simulink model "gm_HDLRx_vs"  (R2024a)
settings: Solver=FixedStepDiscrete  StartTime=0.0  StopTime=stopTime  RelTol=1e-3
undefined symbols (not defined in the file or in its folder): channelBitsPerSubcarrier, channelCyclicPrefixLen, channelOFDMSamples, channelScramblerInit, clk, clk_enable, decimatorDelay, decimatorFilter, fPHY, fs, headerBitsPerFec, headerBitsPerSubcarrier, headerCyclicPrefixLen, headerOFDMSamples, headerScramblerInit, lowerbound, N, numDataCarriers, payloadBitsPerFec, payloadScramblerInit, preambleBitsPerSubcarrier, preambleCyclicPrefixLen, preambleFirstPartOFDMSamples, preambleScramblerInit, preambleSecondPartOFDMSamples, QAM, reset_x, upperbound
libraries: hdlsllib x133, hdlmdlgenlib x132, simulink x8, whdlutilities x8, whdlmod x4, dspsrcs4 x2, whdledac x2, commhdlcrc x1, dsphdlfiltering2 x1, dsphdlsigops2 x1, vivadosimlib x1, HDL_ieee_8021513 x1
(part 3 of 4)

== system gm_HDLRx_vs/full_rx/h_rx_full/h_separate/Compare To Constant ==
  u : Inport  OutDataTypeStr=fixdt(0, 5, 0)  SampleTime=8e-08
  Compare : RelationalOperator  Operator===  OutDataTypeStr=boolean
  Constant : Constant  DisableCoverage=on  Value=const  OutDataTypeStr=fixdt(0, 5, 0)  SampleTime=-1
  y : Outport  SampleTime=8e-08
  wires:
  Constant/1 -> Compare/2
  Compare/1 -> y/1
  u/1 -> Compare/1

== system gm_HDLRx_vs/full_rx/h_rx_full/h_separate/Compare To Constant1 ==
  u : Inport  OutDataTypeStr=fixdt(0, 5, 0)  SampleTime=8e-08
  Compare : RelationalOperator  Operator===  OutDataTypeStr=boolean
  Constant : Constant  DisableCoverage=on  Value=const  OutDataTypeStr=fixdt(0, 5, 0)  SampleTime=-1
  y : Outport  SampleTime=8e-08
  wires:
  Constant/1 -> Compare/2
  Compare/1 -> y/1
  u/1 -> Compare/1

== system gm_HDLRx_vs/full_rx/h_rx_full/h_separate/Compare To Constant2 ==
  u : Inport  OutDataTypeStr=fixdt(0, 5, 0)  SampleTime=8e-08
  Compare : RelationalOperator  Operator===  OutDataTypeStr=boolean
  Constant : Constant  DisableCoverage=on  Value=const  OutDataTypeStr=fixdt(0, 5, 0)  SampleTime=-1
  y : Outport  SampleTime=8e-08
  wires:
  Constant/1 -> Compare/2
  Compare/1 -> y/1
  u/1 -> Compare/1

== system gm_HDLRx_vs/full_rx/h_rx_full/h_separate/Compare To Constant3 ==
  u : Inport  OutDataTypeStr=fixdt(0, 5, 0)  SampleTime=8e-08
  Compare : RelationalOperator  Operator===  OutDataTypeStr=boolean
  Constant : Constant  DisableCoverage=on  Value=const  OutDataTypeStr=fixdt(0, 5, 0)  SampleTime=-1
  y : Outport  SampleTime=8e-08
  wires:
  Constant/1 -> Compare/2
  Compare/1 -> y/1
  u/1 -> Compare/1

== system gm_HDLRx_vs/full_rx/h_rx_full/h_separate/Compare To Constant4 ==
  u : Inport  OutDataTypeStr=fixdt(0, 5, 0)  SampleTime=8e-08
  Compare : RelationalOperator  Operator===  OutDataTypeStr=boolean
  Constant : Constant  DisableCoverage=on  Value=const  OutDataTypeStr=fixdt(0, 5, 0)  SampleTime=-1
  y : Outport  SampleTime=8e-08
  wires:
  Constant/1 -> Compare/2
  Compare/1 -> y/1
  u/1 -> Compare/1

== system gm_HDLRx_vs/full_rx/h_rx_full/h_separate/Compare To Constant5 ==
  u : Inport  OutDataTypeStr=fixdt(0, 5, 0)  SampleTime=8e-08
  Compare : RelationalOperator  Operator===  OutDataTypeStr=boolean
  Constant : Constant  DisableCoverage=on  Value=const  OutDataTypeStr=fixdt(0, 5, 0)  SampleTime=-1
  y : Outport  SampleTime=8e-08
  wires:
  Constant/1 -> Compare/2
  Compare/1 -> y/1
  u/1 -> Compare/1

== system gm_HDLRx_vs/full_rx/h_rx_full/h_separate/Compare To Constant6 ==
  u : Inport  OutDataTypeStr=fixdt(0, 5, 0)  SampleTime=8e-08
  Compare : RelationalOperator  Operator===  OutDataTypeStr=boolean
  Constant : Constant  DisableCoverage=on  Value=const  OutDataTypeStr=fixdt(0, 5, 0)  SampleTime=-1
  y : Outport  SampleTime=8e-08
  wires:
  Constant/1 -> Compare/2
  Compare/1 -> y/1
  u/1 -> Compare/1

== system gm_HDLRx_vs/full_rx/rx_demodulator_full/constellation_descrambler/rising_edge_detector ==
  In : Inport  OutDataTypeStr=boolean  SampleTime=2e-08
  Delay2 : Delay  DelayLength=1  InitialCondition=0  UseCircularBuffer=on
  Logical Operator1 : Logic  IconShape=distinctive  AllPortsSameDT=off  OutDataTypeStr=boolean
  Logical Operator2 : Logic  Operator=NOT  IconShape=distinctive  AllPortsSameDT=off  OutDataTypeStr=boolean
  Out : Outport  SampleTime=2e-08
  wires:
  Logical Operator2/1 -> Logical Operator1/2
  Logical Operator1/1 -> Out/1
  Delay2/1 -> Logical Operator2/1
  In/1 -> Delay2/1, Logical Operator1/1

== system gm_HDLRx_vs/full_rx/rx_demodulator_full/constellation_descrambler/rotate_-90 ==
  data_in : Inport  OutDataTypeStr=fixdt(1, 24, 12)  PortDimensions=1  SampleTime=2e-08
      settings: SignalType=complex
  valid_in : Inport  Port=2  OutDataTypeStr=boolean  PortDimensions=1  SampleTime=2e-08
  s1_in : Inport  Port=3  OutDataTypeStr=boolean  PortDimensions=1  SampleTime=2e-08
  s2_in : Inport  Port=4  OutDataTypeStr=boolean  PortDimensions=1  SampleTime=2e-08
  Delay : Delay  InitialCondition=0  UseCircularBuffer=on
  Delay1 : Delay  InitialCondition=0  UseCircularBuffer=on
  Delay2 : Delay  DelayLength=1  InitialCondition=0  UseCircularBuffer=on
  Delay3 : Delay  DelayLength=1  InitialCondition=0  UseCircularBuffer=on
  rotate_-90 : Subsystem
  data_out : Outport  SampleTime=2e-08  VectorParamsAs1DForOutWhenUnconnected=off
  valid_out : Outport  Port=2  SampleTime=2e-08  VectorParamsAs1DForOutWhenUnconnected=off
  wires:
  rotate_-90/1(data_out) -> Delay2/1
  Delay3/1 -> valid_out/1
  Delay2/1 -> data_out/1
  Delay1/1 -> Delay3/1
  Delay/1 -> rotate_-90/3(data_in)
  s2_in/1 -> rotate_-90/1(s2)
  s1_in/1 -> rotate_-90/2(s1)
  valid_in/1 -> Delay1/1
  data_in/1 -> Delay/1

== system gm_HDLRx_vs/full_rx/rx_demodulator_full/constellation_descrambler/sync_constellation_scrambler ==
  new_ofdm_symbol : Inport  OutDataTypeStr=boolean  SampleTime=2e-08
  init : Inport  Port=2  OutDataTypeStr=boolean  PortDimensions=[13]  SampleTime=2e-08
  valid_in : Inport  Port=3  OutDataTypeStr=boolean  SampleTime=2e-08
  Rate Transition : RateTransition  OutPortSampleTime=1/fPHY
  Rate Transition1 : RateTransition  OutPortSampleTime=1/fPHY
  Rate Transition2 : RateTransition  OutPortSampleTime=1/(2*fPHY)
  Rate Transition3 : RateTransition  OutPortSampleTime=1/(2*fPHY)
  Rate Transition4 : RateTransition  OutPortSampleTime=1/(2*fPHY)
  Synchronous constellation scrambler : Subsystem
  s1 : Outport  SampleTime=2e-08
  s2 : Outport  Port=2  SampleTime=2e-08
  wires:
  Synchronous constellation scrambler/2(s2_out) -> Rate Transition/1
  Synchronous constellation scrambler/1(s1_out) -> Rate Transition1/1
  Rate Transition4/1 -> Synchronous constellation scrambler/1(valid_in)
  Rate Transition3/1 -> Synchronous constellation scrambler/2(init)
  Rate Transition2/1 -> Synchronous constellation scrambler/3(new_ofdm_symbol)
  Rate Transition1/1 -> s1/1
  Rate Transition/1 -> s2/1
  valid_in/1 -> Rate Transition4/1
  init/1 -> Rate Transition3/1
  new_ofdm_symbol/1 -> Rate Transition2/1

== system gm_HDLRx_vs/full_rx/rx_demodulator_full/decimator/rising_edge_detector ==
  In : Inport  OutDataTypeStr=boolean  SampleTime=1e-08
  Delay2 : Delay  DelayLength=1  InitialCondition=0  UseCircularBuffer=on
  Logical Operator1 : Logic  IconShape=distinctive  AllPortsSameDT=off  OutDataTypeStr=boolean
  Logical Operator2 : Logic  Operator=NOT  IconShape=distinctive  AllPortsSameDT=off  OutDataTypeStr=boolean
  Out : Outport  SampleTime=1e-08
  wires:
  Logical Operator2/1 -> Logical Operator1/2
  Logical Operator1/1 -> Out/1
  Delay2/1 -> Logical Operator2/1
  In/1 -> Delay2/1, Logical Operator1/1

== system gm_HDLRx_vs/full_rx/rx_demodulator_full/downshifter/digital_carrier_receiver ==
  dataIn : Inport  OutDataTypeStr=fixdt(1, 16, 12)  PortDimensions=1  SampleTime=1e-08
  ncoIn : Inport  Port=2  OutDataTypeStr=fixdt(1, 16, 12)  PortDimensions=1  SampleTime=1e-08
      settings: SignalType=complex
  Complex to Real-Imag : ComplexToRealImag
  Constant : Constant  Value=2  OutDataTypeStr=fixdt(1, 16, 12)  SampleTime=-1
  Delay{,1..4} (5 alike) : Delay  InitialCondition=0  UseCircularBuffer=on
  Product : Product  OutDataTypeStr=fixdt(1, 16, 12)
  Product1 : Product  InputSameDT=on  OutDataTypeStr=fixdt(1, 16, 12)
  Product2 : Product  OutDataTypeStr=fixdt(1, 16, 12)
  Real-Imag to Complex : RealImagToComplex
  Unary Minus : UnaryMinus
  data_out : Outport  SampleTime=1e-08  VectorParamsAs1DForOutWhenUnconnected=off
  wires:
  Unary Minus/1 -> Delay3/1
  Real-Imag to Complex/1 -> data_out/1
  Product2/1 -> Delay4/1
  Product1/1 -> Delay2/1
  Product/1 -> Delay/1
  Delay4/1 -> Real-Imag to Complex/2
  Delay3/1 -> Product2/1
  Delay2/1 -> Complex to Real-Imag/1
  Delay1/1 -> Product/1
  Delay/1 -> Real-Imag to Complex/1
  Constant/1 -> Product1/1
  Complex to Real-Imag/2 -> Product2/2
  Complex to Real-Imag/1 -> Product/2
  ncoIn/1 -> Product1/2
  dataIn/1 -> Delay1/1, Unary Minus/1

== system gm_HDLRx_vs/full_rx/rx_demodulator_full/downshifter/rising_edge_detector ==
  In : Inport  OutDataTypeStr=boolean  SampleTime=1e-08
  Delay2 : Delay  DelayLength=1  InitialCondition=0  UseCircularBuffer=on
  Logical Operator1 : Logic  IconShape=distinctive  AllPortsSameDT=off  OutDataTypeStr=boolean
  Logical Operator2 : Logic  Operator=NOT  IconShape=distinctive  AllPortsSameDT=off  OutDataTypeStr=boolean
  Out : Outport  SampleTime=1e-08
  wires:
  Logical Operator2/1 -> Logical Operator1/2
  Logical Operator1/1 -> Out/1
  Delay2/1 -> Logical Operator2/1
  In/1 -> Delay2/1, Logical Operator1/1

== system gm_HDLRx_vs/full_rx/rx_demodulator_full/ofdm_rx_counter/falling_edge_detector1 ==
  in : Inport  OutDataTypeStr=boolean  SampleTime=2e-08
  Delay : Delay  DelayLength=1  InitialCondition=0  UseCircularBuffer=on
  Logical Operator : Logic  IconShape=distinctive  AllPortsSameDT=off  OutDataTypeStr=boolean
  Logical Operator1 : Logic  Operator=NOT  IconShape=distinctive  AllPortsSameDT=off  OutDataTypeStr=boolean
  out : Outport  SampleTime=2e-08
  wires:
  Logical Operator1/1 -> Logical Operator/1
  Logical Operator/1 -> out/1
  Delay/1 -> Logical Operator/2
  in/1 -> Delay/1, Logical Operator1/1

== system gm_HDLRx_vs/full_rx/rx_demodulator_full/ofdm_rx_counter/rising_edge_detector1 ==
  In : Inport  OutDataTypeStr=boolean  SampleTime=2e-08
  Delay2 : Delay  DelayLength=1  InitialCondition=0  UseCircularBuffer=on
  Logical Operator1 : Logic  IconShape=distinctive  AllPortsSameDT=off  OutDataTypeStr=boolean
  Logical Operator2 : Logic  Operator=NOT  IconShape=distinctive  AllPortsSameDT=off  OutDataTypeStr=boolean
  Out : Outport  SampleTime=2e-08
  wires:
  Logical Operator2/1 -> Logical Operator1/2
  Logical Operator1/1 -> Out/1
  Delay2/1 -> Logical Operator2/1
  In/1 -> Delay2/1, Logical Operator1/1

== system gm_HDLRx_vs/full_rx/rx_demodulator_full/ofdm_separator/Real Divide HDL Optimized ==
  num : Inport  OutDataTypeStr=fixdt(0, 24, 0)  SampleTime=2e-08
  den : Inport  Port=2  OutDataTypeStr=uint16  SampleTime=2e-08
  validIn : Inport  Port=3  OutDataTypeStr=boolean  SampleTime=2e-08
  Delay17 : Delay  DelayLength=1
  ForEach - Real Divide_instance1 : Subsystem
  Reshape to original size : Subsystem
  Verify divide sizes : Subsystem
  y : Outport  SampleTime=2e-08
  wires:
  Verify divide sizes/2(num) -> ForEach - Real Divide_instance1/2(num)
  Verify divide sizes/1(den) -> ForEach - Real Divide_instance1/1(den)
  Reshape to original size/1(z) -> Delay17/1
  ForEach - Real Divide_instance1/1(y) -> Reshape to original size/1(y)
  Delay17/1 -> y/1
  validIn/1 -> ForEach - Real Divide_instance1/3(validIn)
  den/1 -> Verify divide sizes/1(denominator)
  num/1 -> Reshape to original size/2(u), Verify divide sizes/2(numerator)

== system gm_HDLRx_vs/full_rx/rx_demodulator_full/ofdm_separator/rising_edge_detector ==
  In : Inport  OutDataTypeStr=boolean  SampleTime=2e-08
  Delay2 : Delay  DelayLength=1  InitialCondition=0  UseCircularBuffer=on
  Logical Operator1 : Logic  IconShape=distinctive  AllPortsSameDT=off  OutDataTypeStr=boolean
  Logical Operator2 : Logic  Operator=NOT  IconShape=distinctive  AllPortsSameDT=off  OutDataTypeStr=boolean
  Out : Outport  SampleTime=2e-08
  wires:
  Logical Operator2/1 -> Logical Operator1/2
  Logical Operator1/1 -> Out/1
  Delay2/1 -> Logical Operator2/1
  In/1 -> Delay2/1, Logical Operator1/1

== system gm_HDLRx_vs/full_rx/rx_demodulator_full/qam_demod/to_12bit_integer ==
  1bit : Inport  OutDataTypeStr=fixdt(1, 28, 12)  PortDimensions=1  SampleTime=2e-08
  2bit : Inport  Port=2  OutDataTypeStr=fixdt(1, 28, 12)  PortDimensions=[2 1]  SampleTime=2e-08
  4bit : Inport  Port=3  OutDataTypeStr=fixdt(1, 28, 12)  PortDimensions=[4 1]  SampleTime=2e-08
  Constant{,1..2,12,14} (5 alike) : Constant  Value=0  OutDataTypeStr=fixdt(1, 28, 12)  SampleTime=2e-08
  concatenate : Concatenate  NumInputs=4  Mode=Multidimensional array
  concatenate1 : Concatenate  NumInputs=4  Mode=Multidimensional array
  t : Demux  Outputs=2
  1bit_out : Outport  SampleTime=2e-08
  2bit_out : Outport  Port=2  SampleTime=2e-08
  4bit_out : Outport  Port=3  SampleTime=2e-08
  wires:
  t/2 -> concatenate/4
  t/1 -> concatenate/3
  concatenate1/1 -> 1bit_out/1
  concatenate/1 -> 2bit_out/1
  Constant2/1 -> concatenate1/1
  Constant14/1 -> concatenate/1
  Constant12/1 -> concatenate/2
  Constant1/1 -> concatenate1/2
  Constant/1 -> concatenate1/3
  4bit/1 -> 4bit_out/1
  2bit/1 -> t/1
  1bit/1 -> concatenate1/4

== system gm_HDLRx_vs/full_rx/rx_payload_full/next_frame_to_ready_rx/rising_edge_detector ==
  In : Inport  OutDataTypeStr=boolean  SampleTime=1e-08
  Delay2 : Delay  DelayLength=1  InitialCondition=0  UseCircularBuffer=on
  Logical Operator1 : Logic  IconShape=distinctive  AllPortsSameDT=off  OutDataTypeStr=boolean
  Logical Operator2 : Logic  Operator=NOT  IconShape=distinctive  AllPortsSameDT=off  OutDataTypeStr=boolean
  Out : Outport  SampleTime=1e-08
  wires:
  Logical Operator2/1 -> Logical Operator1/2
  Logical Operator1/1 -> Out/1
  Delay2/1 -> Logical Operator2/1
  In/1 -> Delay2/1, Logical Operator1/1

== system gm_HDLRx_vs/full_rx/rx_payload_full/remove_tone_mapping/valid_to_ctrl ==
  validIn : Inport  OutDataTypeStr=boolean  SampleTime=1e-08
  Delay1 : Delay  DelayLength=1  InitialCondition=0  UseCircularBuffer=on
  Delay2 : Delay  DelayLength=1  InitialCondition=0  UseCircularBuffer=on
  Logical Operator : Logic  IconShape=distinctive  AllPortsSameDT=off  OutDataTypeStr=boolean
  Logical Operator1 : Logic  Operator=NOT  IconShape=distinctive  AllPortsSameDT=off  OutDataTypeStr=boolean
  Logical Operator2 : Logic  IconShape=distinctive  AllPortsSameDT=off  OutDataTypeStr=boolean
  Logical Operator3 : Logic  Operator=NOT  IconShape=distinctive  AllPortsSameDT=off  OutDataTypeStr=boolean
  Sample Control Bus Creator : whdlutilities/Sample Control Bus Creator
  ctrlOut : Outport  SampleTime=1e-08
  wires:
  Sample Control Bus Creator/1 -> ctrlOut/1
  Logical Operator3/1 -> Logical Operator2/2
  Logical Operator2/1 -> Sample Control Bus Creator/2
  Logical Operator1/1 -> Logical Operator/2
  Logical Operator/1 -> Sample Control Bus Creator/1
  Delay2/1 -> Logical Operator1/1
  Delay1/1 -> Sample Control Bus Creator/3, Delay2/1, Logical Operator/1, Logical Operator2/1
  validIn/1 -> Delay1/1, Logical Operator3/1

== system gm_HDLRx_vs/full_rx/rx_demodulator_full/constellation_descrambler/rotate_-90/rotate_-90 ==
  s2 : Inport  OutDataTypeStr=boolean  PortDimensions=1  SampleTime=2e-08
  s1 : Inport  Port=2  OutDataTypeStr=boolean  PortDimensions=1  SampleTime=2e-08
  data_in : Inport  Port=3  OutDataTypeStr=fixdt(1, 24, 12)  PortDimensions=1  SampleTime=2e-08
      settings: SignalType=complex
  Bit Concat : hdlsllib/Logic and Bit Operations/Bit Concat  numInputs=2
  Complex to Real-Imag : ComplexToRealImag
  Complex to Real-Imag1 : ComplexToRealImag
  Complex to Real-Imag2 : ComplexToRealImag
  Multiport Switch : MultiPortSwitch  DataPortOrder=Zero-based contiguous  Inputs=4  zeroidx=on  OutDataTypeStr=fixdt(1, 24, 12)  SaturateOnIntegerOverflow=off  InputSameDT=off
  Real-Imag to Complex : RealImagToComplex
  Real-Imag to Complex1 : RealImagToComplex
  Real-Imag to Complex2 : RealImagToComplex
  Unary Minus{,1..3} (4 alike) : UnaryMinus
  data_out : Outport  SampleTime=2e-08
  wires:
  Unary Minus3/1 -> Real-Imag to Complex/2
  Unary Minus2/1 -> Real-Imag to Complex2/1
  Unary Minus1/1 -> Real-Imag to Complex1/2
  Unary Minus/1 -> Real-Imag to Complex/1
  Real-Imag to Complex2/1 -> Multiport Switch/5
  Real-Imag to Complex1/1 -> Multiport Switch/3
  Real-Imag to Complex/1 -> Multiport Switch/4
  Multiport Switch/1 -> data_out/1
  Complex to Real-Imag2/2 -> Unary Minus2/1
  Complex to Real-Imag2/1 -> Real-Imag to Complex2/2
  Complex to Real-Imag1/2 -> Real-Imag to Complex1/1
  Complex to Real-Imag1/1 -> Unary Minus1/1
  Complex to Real-Imag/2 -> Unary Minus3/1
  Complex to Real-Imag/1 -> Unary Minus/1
  Bit Concat/1 -> Multiport Switch/1
  data_in/1 -> Complex to Real-Imag/1, Complex to Real-Imag1/1, Complex to Real-Imag2/1, Multiport Switch/2
  s1/1 -> Bit Concat/2
  s2/1 -> Bit Concat/1

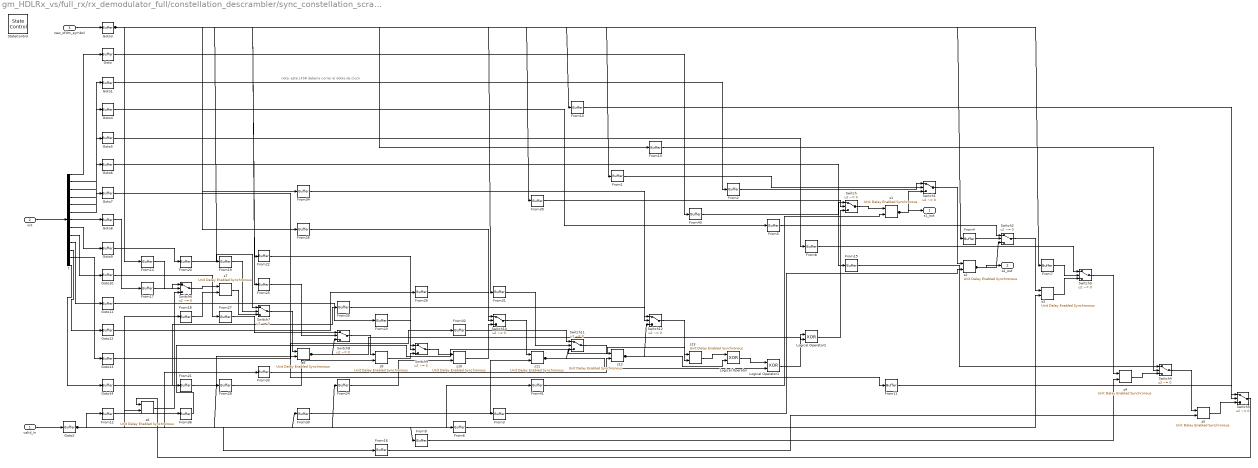
== system gm_HDLRx_vs/full_rx/rx_demodulator_full/constellation_descrambler/sync_constellation_scrambler/Synchronous constellation scrambler ==
  note: nota: este LFSR deberia correr al doble de clock
  valid_in : Inport  OutDataTypeStr=boolean  PortDimensions=1  SampleTime=1e-08
  init : Inport  Port=2  OutDataTypeStr=boolean  PortDimensions=[13]  SampleTime=1e-08
  new_ofdm_symbol : Inport  Port=3  OutDataTypeStr=boolean  PortDimensions=1  SampleTime=1e-08
  From{1..36,39..41} (39 alike) : hdlmdlgenlib/Buffer
  Goto{,1..14} (15 alike) : hdlmdlgenlib/Buffer
  Logical Operator : Logic  Operator=XOR  AllPortsSameDT=off  OutDataTypeStr=boolean  SampleTime=1e-08
  Logical Operator1 : Logic  Operator=XOR  AllPortsSameDT=off  OutDataTypeStr=boolean  SampleTime=1e-08
  Logical Operator2 : Logic  Operator=XOR  AllPortsSameDT=off  OutDataTypeStr=boolean  SampleTime=1e-08
  StateControl : StateControl  StateControl=Synchronous
  Switch{,1..12} (13 alike) : Switch  Criteria=u2 ~= 0  Threshold=double(0)  OutDataTypeStr=boolean  SampleTime=1e-08  SaturateOnIntegerOverflow=off  InputSameDT=off
  s{1..13} (13 alike) : hdlsllib/Discrete/Unit Delay Enabled Synchronous  InitialCondition=double(0)  SampleTime=-1
  t : Demux  Outputs=13
  s1_out : Outport  SampleTime=1e-08  VectorParamsAs1DForOutWhenUnconnected=off
  s2_out : Outport  Port=2  SampleTime=1e-08  VectorParamsAs1DForOutWhenUnconnected=off
  wires:
  t/13 -> Goto14/1
  t/12 -> Goto13/1
  t/11 -> Goto12/1
  t/10 -> Goto11/1
  t/9 -> Goto10/1
  t/8 -> Goto9/1
  t/7 -> Goto8/1
  t/6 -> Goto7/1
  t/5 -> Goto6/1
  t/4 -> Goto5/1
  t/3 -> Goto4/1
  t/2 -> Goto1/1
  t/1 -> Goto/1
  Goto5/1 -> From8/1
  Goto4/1 -> From5/1
  Goto/1 -> From40/1
  Goto14/1 -> From35/1
  Goto13/1 -> From32/1
  Goto12/1 -> From29/1
  Goto10/1 -> From27/1
  Goto11/1 -> From23/1
  Goto9/1 -> From20/1
  Goto1/1 -> From2/1
  Goto8/1 -> From17/1
  Goto6/1 -> From15/1
  Goto2/1 -> From12/1, From16/1, From18/1, From21/1, From24/1, From28/1, From3/1, From30/1, From33/1, From36/1, From41/1, From6/1, From9/1
  Goto7/1 -> From11/1
  Goto3/1 -> From1/1, From10/1, From13/1, From14/1, From19/1, From22/1, From25/1, From26/1, From31/1, From34/1, From39/1, From4/1, From7/1
  s9/1 -> Switch9/3
  s8/1 -> Logical Operator2/2, Switch8/3
  s7/1 -> Switch7/3
  s6/1 -> Switch6/3
  s5/1 -> Switch5/3
  s4/1 -> Switch4/3
  s3/1 -> Switch3/3
  s2/1 -> s2_out/1, Switch2/3
  s13/1 -> Logical Operator/1
  s12/1 -> Logical Operator/2, Switch12/3
  s11/1 -> Logical Operator1/2, Switch11/3
  s10/1 -> Switch10/3
  s1/1 -> s1_out/1, Switch1/3
  Switch9/1 -> s10/1
  Switch8/1 -> s9/1
  Switch7/1 -> s8/1
  Switch6/1 -> s7/1
  Switch5/1 -> s6/1
  Switch4/1 -> s5/1
  Switch3/1 -> s4/1
  Switch2/1 -> s3/1
  Switch12/1 -> s13/1
  Switch11/1 -> s12/1
  Switch10/1 -> s11/1
  Switch1/1 -> s2/1
  Switch/1 -> s1/1
  Logical Operator2/1 -> Switch/3
  Logical Operator1/1 -> Logical Operator2/1
  Logical Operator/1 -> Logical Operator1/1
  From9/1 -> s4/2
  From8/1 -> Switch3/1
  From7/1 -> Switch3/2
  From6/1 -> s3/2
  From5/1 -> Switch2/1
  From41/1 -> s1/2
  From40/1 -> Switch/1
  From4/1 -> Switch2/2
  From39/1 -> Switch/2
  From36/1 -> s13/2
  From35/1 -> Switch12/1
  From34/1 -> Switch12/2
  From33/1 -> s12/2
  From32/1 -> Switch11/1
  From31/1 -> Switch11/2
  From30/1 -> s11/2
  From3/1 -> s2/2
  From29/1 -> Switch10/1
  From28/1 -> s9/2
  From27/1 -> Switch8/1
  From26/1 -> Switch10/2
  From25/1 -> Switch8/2
  From24/1 -> s10/2
  From23/1 -> Switch9/1
  From22/1 -> Switch9/2
  From21/1 -> s8/2
  From20/1 -> Switch7/1
  From2/1 -> Switch1/1
  From19/1 -> Switch7/2
  From18/1 -> s7/2
  From17/1 -> Switch6/1
  From16/1 -> s5/2
  From15/1 -> Switch4/1
  From14/1 -> Switch6/2
  From13/1 -> Switch4/2
  From12/1 -> s6/2
  From11/1 -> Switch5/1
  From10/1 -> Switch5/2
  From1/1 -> Switch1/2
  new_ofdm_symbol/1 -> Goto3/1
  init/1 -> t/1
  valid_in/1 -> Goto2/1

== system gm_HDLRx_vs/full_rx/rx_demodulator_full/ofdm_separator/Real Divide HDL Optimized/ForEach - Real Divide_instance1 ==
  note: For Each
  den : Inport  OutDataTypeStr=uint16  PortDimensions=1  SampleTime=2e-08
  num : Inport  Port=2  OutDataTypeStr=fixdt(0, 24, 0)  PortDimensions=1  SampleTime=2e-08
  validIn : Inport  Port=3  OutDataTypeStr=boolean  PortDimensions=1  SampleTime=2e-08
  Delay{1,4,14..17,25..26} (8 alike) : Delay  DelayLength=1
  Delay{2,9..12,18} (6 alike) : Delay
  Divide by zero handler : Subsystem
  Divide real numerator by denominator : Subsystem
  MATLAB Function : Subsystem
  Normalize denominator : Subsystem  mask(Real Normalizer HDL Optimized){}
      mask help: fixed:emblib:RealNormalizerFullDescription
      mask Help: For internal use only. This feature is intentionally undocumented. Its behavior may change, or it may be removed in a future release.
      mask Display:
      | text(0.5,0.8,'u ~= 0','texmode','on','HorizontalAlignment','center')
      | text(0.5,0.6,'x = 2^e |u|','texmode','on','HorizontalAlignment','center')
      | text(0.5,0.4,'1 \leq x < 2','texmode','on','HorizontalAlignment','center')
      | text(0.5,0.2,'isNegative = u<0','texmode','on','HorizontalAlignment','center')
  Normalize numerator : Subsystem  mask(Real Normalizer HDL Optimized){}
      mask help: fixed:emblib:RealNormalizerFullDescription
      mask Help: For internal use only. This feature is intentionally undocumented. Its behavior may change, or it may be removed in a future release.
      mask Display:
      | text(0.5,0.8,'u ~= 0','texmode','on','HorizontalAlignment','center')
      | text(0.5,0.6,'x = 2^e |u|','texmode','on','HorizontalAlignment','center')
      | text(0.5,0.4,'1 \leq x < 2','texmode','on','HorizontalAlignment','center')
      | text(0.5,0.2,'isNegative = u<0','texmode','on','HorizontalAlignment','center')
  Shift and cast to output type : Subsystem  mask{OutputType=OutputType}
      mask prompts: OutputType "fixed:emblib:OutputPrototype"
  Switch : Switch  Criteria=u2 ~= 0  OutDataTypeStr=int16  SaturateOnIntegerOverflow=off  InputSameDT=off
  Unit Delay Enabled Synchronous : hdlsllib/Discrete/Unit Delay Enabled Synchronous  InitialCondition=0.0  SampleTime=-1
  Unit Delay Enabled Synchronous1 : hdlsllib/Discrete/Unit Delay Enabled Synchronous  InitialCondition=0.0  SampleTime=-1
  Unit Delay Enabled Synchronous2 : hdlsllib/Discrete/Unit Delay Enabled Synchronous  InitialCondition=0.0  SampleTime=-1
      settings: LibrarySourceBlock=|
      | embreciprocals/Real Divide HDL Optimized/ForEach - Real Divide/Unit Delay Enabled
      | Synchronous1
  Upcast Wordlength : Subsystem
  y : Outport  SampleTime=2e-08
  wires:
  Delay1/1 -> y/1
  Delay10/1 -> Divide real numerator by denominator/4(tDen)
  Delay11/1 -> Divide real numerator by denominator/6(isDenNegative)
  Delay12/1 -> Divide real numerator by denominator/7(validIn)
  Delay14/1 -> Normalize numerator/1(u)
  Delay15/1 -> Normalize numerator/2(validIn), Normalize denominator/2(validIn)
  Delay16/1 -> Divide real numerator by denominator/1(num)
  Delay17/1 -> Divide real numerator by denominator/2(tNum)
  Delay18/1 -> Divide real numerator by denominator/5(isNumNegative)
  Delay2/1 -> Switch/2
  Delay25/1 -> MATLAB Function/1(num)
  Delay26/1 -> MATLAB Function/2(t_num)
  Delay4/1 -> Normalize denominator/1(u)
  Delay9/1 -> Divide real numerator by denominator/3(den)
  Divide by zero handler/1(yOut) -> Switch/1
  Divide real numerator by denominator/4(validOut) -> Unit Delay Enabled Synchronous2/2, Unit Delay Enabled Synchronous1/2, Unit Delay Enabled Synchronous/2
  Divide real numerator by denominator/3(isDenZero) -> Unit Delay Enabled Synchronous2/1
  Divide real numerator by denominator/2(e) -> Unit Delay Enabled Synchronous1/1
  Divide real numerator by denominator/1(y) -> Unit Delay Enabled Synchronous/1
  MATLAB Function/2(t_num_out) -> Delay17/1
  MATLAB Function/1(num_out) -> Delay16/1
  Normalize denominator/4(validOut) -> Delay12/1
  Normalize denominator/3(isNegative) -> Delay11/1
  Normalize denominator/2(e) -> Delay10/1
  Normalize denominator/1(x) -> Delay9/1
  Normalize numerator/3(isNegative) -> Delay18/1
  Normalize numerator/2(e) -> Delay26/1
  Normalize numerator/1(x) -> Delay25/1
  Shift and cast to output type/1(y) -> Switch/3
  Switch/1 -> Delay1/1
  Unit Delay Enabled Synchronous/1 -> Shift and cast to output type/1(x), Divide by zero handler/1(yIn)
  Unit Delay Enabled Synchronous1/1 -> Shift and cast to output type/2(shiftValue)
  Unit Delay Enabled Synchronous2/1 -> Delay2/1
  Upcast Wordlength/2(v) -> Delay14/1
  Upcast Wordlength/1(u) -> Delay4/1
  validIn/1 -> Delay15/1
  num/1 -> Upcast Wordlength/2(y)
  den/1 -> Upcast Wordlength/1(x)

== system gm_HDLRx_vs/full_rx/rx_demodulator_full/ofdm_separator/Real Divide HDL Optimized/Reshape to original size ==
  y : Inport  OutDataTypeStr=int16  PortDimensions=1  SampleTime=2e-08
  u : Inport  Port=2  OutDataTypeStr=fixdt(0, 24, 0)  PortDimensions=1  SampleTime=2e-08
  embreciprocals_c11_Reshape_to_original_size : MATLAB Function  TreatAsAtomicUnit=on
      settings: LibrarySourceBlock=embreciprocals/Real Divide HDL Optimized/Reshape to original size
  z : Outport  SampleTime=2e-08
  wires:
  embreciprocals_c11_Reshape_to_original_size/1(z) -> z/1
  u/1 -> embreciprocals_c11_Reshape_to_original_size/2(u)
  y/1 -> embreciprocals_c11_Reshape_to_original_size/1(y)

== system gm_HDLRx_vs/full_rx/rx_demodulator_full/ofdm_separator/Real Divide HDL Optimized/Verify divide sizes ==
  denominator : Inport  OutDataTypeStr=uint16  PortDimensions=1  SampleTime=2e-08
  numerator : Inport  Port=2  OutDataTypeStr=fixdt(0, 24, 0)  PortDimensions=1  SampleTime=2e-08
  embreciprocals_c19_Verify_divide_sizes : MATLAB Function  TreatAsAtomicUnit=on
      settings: LibrarySourceBlock=embreciprocals/Real Divide HDL Optimized/Verify divide sizes
  den : Outport  SampleTime=2e-08
  num : Outport  Port=2  SampleTime=2e-08
  wires:
  embreciprocals_c19_Verify_divide_sizes/2(num) -> num/1
  embreciprocals_c19_Verify_divide_sizes/1(den) -> den/1
  numerator/1 -> embreciprocals_c19_Verify_divide_sizes/2(numerator)
  denominator/1 -> embreciprocals_c19_Verify_divide_sizes/1(denominator)

== system gm_HDLRx_vs/full_rx/rx_demodulator_full/ofdm_separator/Real Divide HDL Optimized/ForEach - Real Divide_instance1/Divide by zero handler ==
  yIn : Inport  OutDataTypeStr=fixdt(1, 25, 23)  SampleTime=2e-08
  Compare To Zero : Subsystem  mask(Compare To Zero){relop=>=, OutDataTypeStr=boolean, ZeroCross=on}
      mask prompts: relop "Simulink:masks:Operator_MP"; OutDataTypeStr "Simulink:masks:OutputDataType_MP"; ZeroCross "Simulink:masks:EnableZerocrossingDetection_MP"
      mask help: Simulink:masks:CompareToZero_MD
      mask init:
      | OutDataTypeStr = 'boolean';
      | ZeroCross = 'on';
      | blkName = 'HDLRx/full_rx/rx_demodulator_full/ofdm_separator/Real Divide HDL Optimized/ForEach - Real Divide/Divide by zero handler/Compare\nTo Zero';
      | relop = '>=';
      | setValue = 'boolean';
      mask TypeOptions relop: == | ~= | < | <= | >= | >
      mask TypeOptions OutDataTypeStr: Simulink:masks:uint8 | Simulink:masks:boolean
      mask Callback ZeroCross: sl('zeroCrossEnable', gcbh);
      mask Display: disp([relop,' 0'])
  Constant3 : Constant  Value=lowerbound(numerictype(OutputType))  OutDataTypeStr=OutputType  SampleTime=-1
  Constant4 : Constant  Value=upperbound(numerictype(OutputType))  OutDataTypeStr=OutputType  SampleTime=-1
  Delay13 : Delay  DelayLength=1
  Delay3 : Delay  DelayLength=1
  Switch : Switch  Criteria=u2 > Threshold  OutDataTypeStr=int16  SaturateOnIntegerOverflow=off  InputSameDT=off
  yOut : Outport  SampleTime=2e-08
  wires:
  yIn/1 -> Compare To Zero/1(u)
  Compare To Zero/1(y) -> Delay13/1
  Constant3/1 -> Switch/3
  Constant4/1 -> Switch/1
  Delay13/1 -> Switch/2
  Delay3/1 -> yOut/1
  Switch/1 -> Delay3/1

== system gm_HDLRx_vs/full_rx/rx_demodulator_full/ofdm_separator/Real Divide HDL Optimized/ForEach - Real Divide_instance1/Divide real numerator by denominator ==
  num : Inport  OutDataTypeStr=fixdt(1, 25, 23)  SampleTime=2e-08
  tNum : Inport  Port=2  OutDataTypeStr=fixdt(1, 33, 0)  SampleTime=2e-08
  den : Inport  Port=3  OutDataTypeStr=fixdt(1, 25, 23)  SampleTime=2e-08
  tDen : Inport  Port=4  OutDataTypeStr=int32  SampleTime=2e-08
  isNumNegative : Inport  Port=5  OutDataTypeStr=boolean  SampleTime=2e-08
  isDenNegative : Inport  Port=6  OutDataTypeStr=boolean  SampleTime=2e-08
  validIn : Inport  Port=7  OutDataTypeStr=boolean  SampleTime=2e-08
  normalizedCORDICDivide : Subsystem
  y : Outport  SampleTime=2e-08
  e : Outport  Port=2  SampleTime=2e-08
  isDenZero : Outport  Port=3  SampleTime=2e-08
  validOut : Outport  Port=4  SampleTime=2e-08
  wires:
  validIn/1 -> normalizedCORDICDivide/7(validIn)
  isDenNegative/1 -> normalizedCORDICDivide/6(isDenNegative)
  isNumNegative/1 -> normalizedCORDICDivide/5(isNumNegative)
  tDen/1 -> normalizedCORDICDivide/4(tDen)
  den/1 -> normalizedCORDICDivide/2(den)
  tNum/1 -> normalizedCORDICDivide/3(tNum)
  num/1 -> normalizedCORDICDivide/1(num)
  normalizedCORDICDivide/4(validOut) -> validOut/1
  normalizedCORDICDivide/3(isDenZeroOut) -> isDenZero/1
  normalizedCORDICDivide/2(t) -> e/1
  normalizedCORDICDivide/1(y) -> y/1

== system gm_HDLRx_vs/full_rx/rx_demodulator_full/ofdm_separator/Real Divide HDL Optimized/ForEach - Real Divide_instance1/MATLAB Function ==
  num : Inport  OutDataTypeStr=fixdt(1, 25, 23)  PortDimensions=1  SampleTime=2e-08
  t_num : Inport  Port=2  OutDataTypeStr=int32  PortDimensions=1  SampleTime=2e-08
  embreciprocals_c13_MATLAB_Function : MATLAB Function  TreatAsAtomicUnit=on
      settings: LibrarySourceBlock=embreciprocals/Real Divide HDL Optimized/ForEach - Real Divide/MATLAB Function
  num_out : Outport  SampleTime=2e-08
  t_num_out : Outport  Port=2  SampleTime=2e-08
  wires:
  embreciprocals_c13_MATLAB_Function/2(t_num_out) -> t_num_out/1
  embreciprocals_c13_MATLAB_Function/1(num_out) -> num_out/1
  t_num/1 -> embreciprocals_c13_MATLAB_Function/2(t_num)
  num/1 -> embreciprocals_c13_MATLAB_Function/1(num)

== system gm_HDLRx_vs/full_rx/rx_demodulator_full/ofdm_separator/Real Divide HDL Optimized/ForEach - Real Divide_instance1/Normalize denominator ==
  u : Inport  OutDataTypeStr=fixdt(1, 25, 8)  SampleTime=2e-08
  validIn : Inport  Port=2  OutDataTypeStr=boolean  SampleTime=2e-08
  positiveRealNormalizer : Subsystem
  x : Outport  SampleTime=2e-08
  e : Outport  Port=2  SampleTime=2e-08
  isNegative : Outport  Port=3  SampleTime=2e-08
  validOut : Outport  Port=4  SampleTime=2e-08
  wires:
  validIn/1 -> positiveRealNormalizer/2(validIn)
  u/1 -> positiveRealNormalizer/1(u)
  positiveRealNormalizer/4(validOut) -> validOut/1
  positiveRealNormalizer/3(isNegative) -> isNegative/1
  positiveRealNormalizer/2(e) -> e/1
  positiveRealNormalizer/1(x) -> x/1

== system gm_HDLRx_vs/full_rx/rx_demodulator_full/ofdm_separator/Real Divide HDL Optimized/ForEach - Real Divide_instance1/Normalize numerator ==
  u : Inport  OutDataTypeStr=fixdt(1, 25, 0)  SampleTime=2e-08
  validIn : Inport  Port=2  OutDataTypeStr=boolean  SampleTime=2e-08
  positiveRealNormalizer : Subsystem
  positiveRealNormalizer_term3 : Terminator
  x : Outport  SampleTime=2e-08
  e : Outport  Port=2  SampleTime=2e-08
  isNegative : Outport  Port=3  SampleTime=2e-08
  wires:
  positiveRealNormalizer/4(validOut) -> positiveRealNormalizer_term3/1
  validIn/1 -> positiveRealNormalizer/2(validIn)
  u/1 -> positiveRealNormalizer/1(u)
  positiveRealNormalizer/3(isNegative) -> isNegative/1
  positiveRealNormalizer/2(e) -> e/1
  positiveRealNormalizer/1(x) -> x/1

== system gm_HDLRx_vs/full_rx/rx_demodulator_full/ofdm_separator/Real Divide HDL Optimized/ForEach - Real Divide_instance1/Shift and cast to output type ==
  x : Inport  OutDataTypeStr=fixdt(1, 25, 23)  SampleTime=2e-08
  shiftValue : Inport  Port=2  OutDataTypeStr=fixdt(1, 34, 0)  SampleTime=2e-08
  Abs : Abs  OutDataTypeStr=fixdt('int32', 'DataTypeOverride', 'Off')  SaturateOnIntegerOverflow=off
  Cast to Union of Types : Subsystem
  Constant : Constant  Value=0  OutDataTypeStr=OutputType  SampleTime=-1
  Data Type Conversion : DataTypeConversion  OutDataTypeStr=OutputType  RndMeth=Floor
  Delay1 : Delay  DelayLength=1
  Delay3 : Delay  DelayLength=1
  Switch : Switch  OutDataTypeStr=fixdt(1, 39, 23)  SaturateOnIntegerOverflow=off  InputSameDT=off
  Variable Left Shift : Subsystem
  Variable Right Shift : Subsystem
  y : Outport  SampleTime=2e-08
  wires:
  shiftValue/1 -> Delay3/1, Abs/1
  x/1 -> Cast to Union of Types/2(Cin)
  Abs/1 -> Variable Right Shift/2(rightShift), Variable Left Shift/2(leftShift)
  Cast to Union of Types/1(Cout) -> Variable Left Shift/1(x), Variable Right Shift/1(x)
  Constant/1 -> Cast to Union of Types/1(Xref)
  Data Type Conversion/1 -> y/1
  Delay1/1 -> Data Type Conversion/1
  Delay3/1 -> Switch/2
  Switch/1 -> Delay1/1
  Variable Left Shift/1(y) -> Switch/1
  Variable Right Shift/1(y) -> Switch/3

== system gm_HDLRx_vs/full_rx/rx_demodulator_full/ofdm_separator/Real Divide HDL Optimized/ForEach - Real Divide_instance1/Upcast Wordlength ==
  x : Inport  OutDataTypeStr=uint16  SampleTime=2e-08
  y : Inport  Port=2  OutDataTypeStr=fixdt(0, 24, 0)  SampleTime=2e-08
  slutils_c2_Upcast_Wordlength : MATLAB Function
      settings: LibrarySourceBlock=slutils/Upcast Wordlength
  u : Outport  SampleTime=2e-08
  v : Outport  Port=2  SampleTime=2e-08
  wires:
  slutils_c2_Upcast_Wordlength/2(v) -> v/1
  slutils_c2_Upcast_Wordlength/1(u) -> u/1
  y/1 -> slutils_c2_Upcast_Wordlength/2(y)
  x/1 -> slutils_c2_Upcast_Wordlength/1(x)

== system gm_HDLRx_vs/full_rx/rx_demodulator_full/ofdm_separator/Real Divide HDL Optimized/ForEach - Real Divide_instance1/Divide by zero handler/Compare To Zero ==
  u : Inport  OutDataTypeStr=fixdt(1, 25, 23)  SampleTime=2e-08
  Compare : RelationalOperator  OutDataTypeStr=boolean
  Constant : Constant  DisableCoverage=on  Value=0  OutDataTypeStr=fixdt(1, 25, 23)  SampleTime=-1  PreserveConstantTs=on
  y : Outport  SampleTime=2e-08
  wires:
  u/1 -> Compare/1
  Compare/1 -> y/1
  Constant/1 -> Compare/2

== system gm_HDLRx_vs/full_rx/rx_demodulator_full/ofdm_separator/Real Divide HDL Optimized/ForEach - Real Divide_instance1/Divide real numerator by denominator/normalizedCORDICDivide ==
  num : Inport  OutDataTypeStr=fixdt(1, 25, 23)  PortDimensions=1  SampleTime=2e-08
  den : Inport  Port=2  OutDataTypeStr=fixdt(1, 25, 23)  PortDimensions=1  SampleTime=2e-08
  tNum : Inport  Port=3  OutDataTypeStr=fixdt(1, 33, 0)  PortDimensions=1  SampleTime=2e-08
  tDen : Inport  Port=4  OutDataTypeStr=int32  PortDimensions=1  SampleTime=2e-08
  isNumNegative : Inport  Port=5  OutDataTypeStr=boolean  PortDimensions=1  SampleTime=2e-08
  isDenNegative : Inport  Port=6  OutDataTypeStr=boolean  PortDimensions=1  SampleTime=2e-08
  validIn : Inport  Port=7  OutDataTypeStr=boolean  PortDimensions=1  SampleTime=2e-08
  embreciprocals_c21_normalizedCORDICDivide : MATLAB Function  TreatAsAtomicUnit=on
      settings: LibrarySourceBlock=embreciprocals/Divide real numerator by denominator/normalizedCORDICDivide
  y : Outport  SampleTime=2e-08  VectorParamsAs1DForOutWhenUnconnected=off
  t : Outport  Port=2  SampleTime=2e-08  VectorParamsAs1DForOutWhenUnconnected=off
  isDenZeroOut : Outport  Port=3  SampleTime=2e-08
  validOut : Outport  Port=4  SampleTime=2e-08  VectorParamsAs1DForOutWhenUnconnected=off
  wires:
  embreciprocals_c21_normalizedCORDICDivide/4(validOut) -> validOut/1
  embreciprocals_c21_normalizedCORDICDivide/3(isDenZeroOut) -> isDenZeroOut/1
  embreciprocals_c21_normalizedCORDICDivide/2(t) -> t/1
  embreciprocals_c21_normalizedCORDICDivide/1(y) -> y/1
  validIn/1 -> embreciprocals_c21_normalizedCORDICDivide/7(validIn)
  isDenNegative/1 -> embreciprocals_c21_normalizedCORDICDivide/6(isDenNegative)
  isNumNegative/1 -> embreciprocals_c21_normalizedCORDICDivide/5(isNumNegative)
  tDen/1 -> embreciprocals_c21_normalizedCORDICDivide/4(tDen)
  tNum/1 -> embreciprocals_c21_normalizedCORDICDivide/3(tNum)
  den/1 -> embreciprocals_c21_normalizedCORDICDivide/2(den)
  num/1 -> embreciprocals_c21_normalizedCORDICDivide/1(num)

== system gm_HDLRx_vs/full_rx/rx_demodulator_full/ofdm_separator/Real Divide HDL Optimized/ForEach - Real Divide_instance1/Normalize denominator/positiveRealNormalizer ==
  u : Inport  OutDataTypeStr=fixdt(1, 25, 8)  PortDimensions=1  SampleTime=2e-08
  validIn : Inport  Port=2  OutDataTypeStr=boolean  PortDimensions=1  SampleTime=2e-08
  embreciprocals_c3_szUwl4UaRWSwHB6ziXbSTrD_positiveRealNormalize : MATLAB Function  TreatAsAtomicUnit=on
      settings: LibrarySourceBlock=embreciprocals/Real Normalizer HDL Optimized/positiveRealNormalizer
  x : Outport  SampleTime=2e-08  VectorParamsAs1DForOutWhenUnconnected=off
  e : Outport  Port=2  SampleTime=2e-08  VectorParamsAs1DForOutWhenUnconnected=off
  isNegative : Outport  Port=3  SampleTime=2e-08
  validOut : Outport  Port=4  SampleTime=2e-08  VectorParamsAs1DForOutWhenUnconnected=off
  wires:
  embreciprocals_c3_szUwl4UaRWSwHB6ziXbSTrD_positiveRealNormalize/4(validOut) -> validOut/1
  embreciprocals_c3_szUwl4UaRWSwHB6ziXbSTrD_positiveRealNormalize/3(isNegative) -> isNegative/1
  embreciprocals_c3_szUwl4UaRWSwHB6ziXbSTrD_positiveRealNormalize/2(e) -> e/1
  embreciprocals_c3_szUwl4UaRWSwHB6ziXbSTrD_positiveRealNormalize/1(x) -> x/1
  validIn/1 -> embreciprocals_c3_szUwl4UaRWSwHB6ziXbSTrD_positiveRealNormalize/2(validIn)
  u/1 -> embreciprocals_c3_szUwl4UaRWSwHB6ziXbSTrD_positiveRealNormalize/1(u)

== system gm_HDLRx_vs/full_rx/rx_demodulator_full/ofdm_separator/Real Divide HDL Optimized/ForEach - Real Divide_instance1/Normalize numerator/positiveRealNormalizer ==
  u : Inport  OutDataTypeStr=fixdt(1, 25, 0)  PortDimensions=1  SampleTime=2e-08
  validIn : Inport  Port=2  OutDataTypeStr=boolean  PortDimensions=1  SampleTime=2e-08
  embreciprocals_c3_s14mscxAahtiBqnXaktE2fE_positiveRealNormalize : MATLAB Function  TreatAsAtomicUnit=on
      settings: LibrarySourceBlock=embreciprocals/Real Normalizer HDL Optimized/positiveRealNormalizer
  embreciprocals_c3_s14mscxAahtiBqnXaktE2fE_positiveRealNormalize_term3 : Terminator
  t : Constant  Value=double(0)  OutDataTypeStr=boolean  SampleTime=2e-08
  x : Outport  SampleTime=2e-08  VectorParamsAs1DForOutWhenUnconnected=off
  e : Outport  Port=2  SampleTime=2e-08  VectorParamsAs1DForOutWhenUnconnected=off
  isNegative : Outport  Port=3  SampleTime=2e-08
  validOut : Outport  Port=4  SampleTime=2e-08  VectorParamsAs1DForOutWhenUnconnected=off
  wires:
  t/1 -> validOut/1
  embreciprocals_c3_s14mscxAahtiBqnXaktE2fE_positiveRealNormalize/4(validOut) -> embreciprocals_c3_s14mscxAahtiBqnXaktE2fE_positiveRealNormalize_term3/1
  embreciprocals_c3_s14mscxAahtiBqnXaktE2fE_positiveRealNormalize/3(isNegative) -> isNegative/1
  embreciprocals_c3_s14mscxAahtiBqnXaktE2fE_positiveRealNormalize/2(e) -> e/1
  embreciprocals_c3_s14mscxAahtiBqnXaktE2fE_positiveRealNormalize/1(x) -> x/1
  validIn/1 -> embreciprocals_c3_s14mscxAahtiBqnXaktE2fE_positiveRealNormalize/2(validIn)
  u/1 -> embreciprocals_c3_s14mscxAahtiBqnXaktE2fE_positiveRealNormalize/1(u)

== system gm_HDLRx_vs/full_rx/rx_demodulator_full/ofdm_separator/Real Divide HDL Optimized/ForEach - Real Divide_instance1/Shift and cast to output type/Cast to Union of Types ==
  Xref : Inport  OutDataTypeStr=int16  SampleTime=2e-08
  Cin : Inport  Port=2  OutDataTypeStr=fixdt(1, 25, 23)  SampleTime=2e-08
  slutils_c1_Cast_to_Union_of_Types : MATLAB Function
      settings: LibrarySourceBlock=slutils/Cast to Union of Types
  Cout : Outport  SampleTime=2e-08
  wires:
  slutils_c1_Cast_to_Union_of_Types/1(Cout) -> Cout/1
  Cin/1 -> slutils_c1_Cast_to_Union_of_Types/2(Cin)
  Xref/1 -> slutils_c1_Cast_to_Union_of_Types/1(Xref)

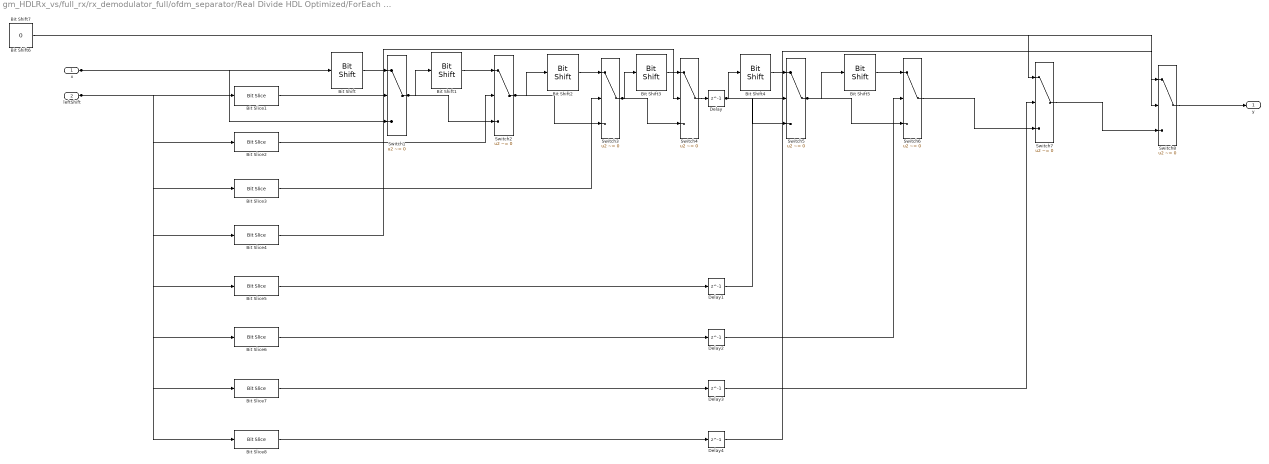
== system gm_HDLRx_vs/full_rx/rx_demodulator_full/ofdm_separator/Real Divide HDL Optimized/ForEach - Real Divide_instance1/Shift and cast to output type/Variable Left Shift ==
  x : Inport  OutDataTypeStr=fixdt(1, 39, 23)  SampleTime=2e-08
  leftShift : Inport  Port=2  OutDataTypeStr=int32  SampleTime=2e-08
  Bit Shift : hdlsllib/Logic and Bit Operations/Bit Shift  mode=Shift Left Logical  N=1
  Bit Shift1 : hdlsllib/Logic and Bit Operations/Bit Shift  mode=Shift Left Logical  N=2
  Bit Shift2 : hdlsllib/Logic and Bit Operations/Bit Shift  mode=Shift Left Logical  N=4
  Bit Shift3 : hdlsllib/Logic and Bit Operations/Bit Shift  mode=Shift Left Logical  N=8
  Bit Shift4 : hdlsllib/Logic and Bit Operations/Bit Shift  mode=Shift Left Logical  N=16
  Bit Shift5 : hdlsllib/Logic and Bit Operations/Bit Shift  mode=Shift Left Logical  N=32
  Bit Shift6 : Constant  Value=0  OutDataTypeStr=fixdt(1, 39, 23)  SampleTime=2e-08
  Bit Shift7 : Constant  Value=0  OutDataTypeStr=fixdt(1, 39, 23)  SampleTime=2e-08
  Bit Slice1 : hdlsllib/Logic and Bit Operations/Bit Slice  lidx=0  ridx=0
      settings: LibrarySourceBlock=embreciprocals/Real Divide HDL Optimized/ForEach - Real Divide/Shift and cast to output type/Variable Left Shift/Bit Slice1
  Bit Slice2 : hdlsllib/Logic and Bit Operations/Bit Slice  lidx=1  ridx=1
      settings: LibrarySourceBlock=embreciprocals/Real Divide HDL Optimized/ForEach - Real Divide/Shift and cast to output type/Variable Left Shift/Bit Slice2
  Bit Slice3 : hdlsllib/Logic and Bit Operations/Bit Slice  lidx=2  ridx=2
      settings: LibrarySourceBlock=embreciprocals/Real Divide HDL Optimized/ForEach - Real Divide/Shift and cast to output type/Variable Left Shift/Bit Slice3
  Bit Slice4 : hdlsllib/Logic and Bit Operations/Bit Slice  lidx=3  ridx=3
      settings: LibrarySourceBlock=embreciprocals/Real Divide HDL Optimized/ForEach - Real Divide/Shift and cast to output type/Variable Left Shift/Bit Slice4
  Bit Slice5 : hdlsllib/Logic and Bit Operations/Bit Slice  lidx=4  ridx=4
      settings: LibrarySourceBlock=embreciprocals/Real Divide HDL Optimized/ForEach - Real Divide/Shift and cast to output type/Variable Left Shift/Bit Slice5
  Bit Slice6 : hdlsllib/Logic and Bit Operations/Bit Slice  lidx=5  ridx=5
      settings: LibrarySourceBlock=embreciprocals/Real Divide HDL Optimized/ForEach - Real Divide/Shift and cast to output type/Variable Left Shift/Bit Slice6
  Bit Slice7 : hdlsllib/Logic and Bit Operations/Bit Slice  lidx=6  ridx=6
      settings: LibrarySourceBlock=embreciprocals/Real Divide HDL Optimized/ForEach - Real Divide/Shift and cast to output type/Variable Left Shift/Bit Slice7
  Bit Slice8 : hdlsllib/Logic and Bit Operations/Bit Slice  lidx=7  ridx=7
      settings: LibrarySourceBlock=embreciprocals/Real Divide HDL Optimized/ForEach - Real Divide/Shift and cast to output type/Variable Left Shift/Bit Slice8
  Delay{,1..4} (5 alike) : Delay  DelayLength=1
  Switch{1..8} (8 alike) : Switch  Criteria=u2 ~= 0  OutDataTypeStr=fixdt(1, 39, 23)  SaturateOnIntegerOverflow=off  InputSameDT=off
  y : Outport  SampleTime=2e-08
  wires:
  leftShift/1 -> Bit Slice8/1, Bit Slice7/1, Bit Slice6/1, Bit Slice5/1, Bit Slice4/1, Bit Slice3/1, Bit Slice2/1, Bit Slice1/1
  x/1 -> Switch1/3, Bit Shift/1
  Bit Shift/1 -> Switch1/1
  Bit Shift1/1 -> Switch2/1
  Bit Shift2/1 -> Switch3/1
  Bit Shift3/1 -> Switch4/1
  Bit Shift4/1 -> Switch5/1
  Bit Shift5/1 -> Switch6/1
  Bit Shift6/1 -> Switch7/1
  Bit Shift7/1 -> Switch8/1
  Bit Slice1/1 -> Switch1/2
  Bit Slice2/1 -> Switch2/2
  Bit Slice3/1 -> Switch3/2
  Bit Slice4/1 -> Switch4/2
  Bit Slice5/1 -> Delay1/1
  Bit Slice6/1 -> Delay2/1
  Bit Slice7/1 -> Delay3/1
  Bit Slice8/1 -> Delay4/1
  Delay/1 -> Switch5/3, Bit Shift4/1
  Delay1/1 -> Switch5/2
  Delay2/1 -> Switch6/2
  Delay3/1 -> Switch7/2
  Delay4/1 -> Switch8/2
  Switch1/1 -> Switch2/3, Bit Shift1/1
  Switch2/1 -> Switch3/3, Bit Shift2/1
  Switch3/1 -> Switch4/3, Bit Shift3/1
  Switch4/1 -> Delay/1
  Switch5/1 -> Switch6/3, Bit Shift5/1
  Switch6/1 -> Switch7/3
  Switch7/1 -> Switch8/3
  Switch8/1 -> y/1

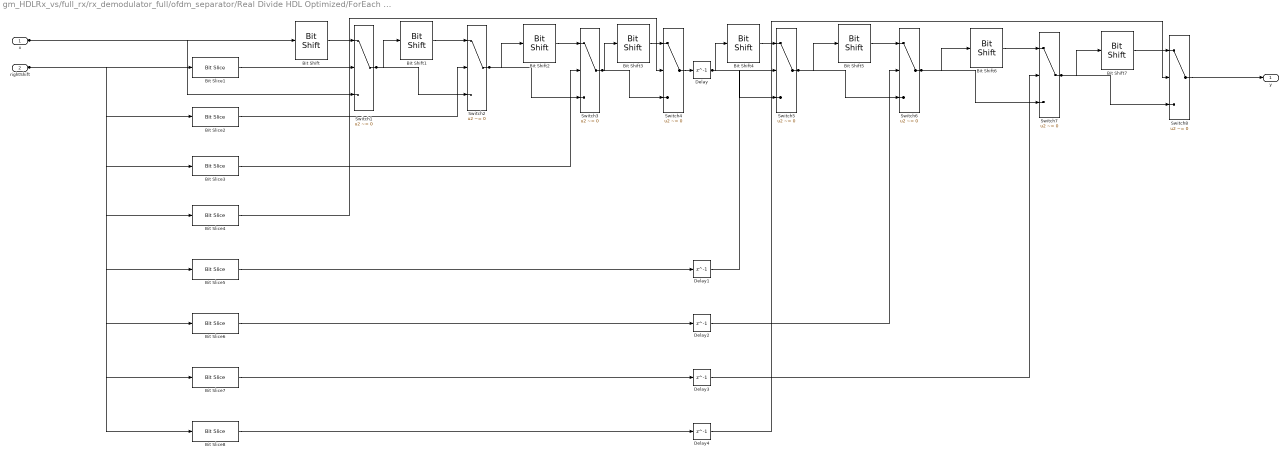
== system gm_HDLRx_vs/full_rx/rx_demodulator_full/ofdm_separator/Real Divide HDL Optimized/ForEach - Real Divide_instance1/Shift and cast to output type/Variable Right Shift ==
  x : Inport  OutDataTypeStr=fixdt(1, 39, 23)  SampleTime=2e-08
  rightShift : Inport  Port=2  OutDataTypeStr=int32  SampleTime=2e-08
  Bit Shift : hdlsllib/Logic and Bit Operations/Bit Shift  mode=Shift Right Arithmetic  N=1
  Bit Shift1 : hdlsllib/Logic and Bit Operations/Bit Shift  mode=Shift Right Arithmetic  N=2
  Bit Shift2 : hdlsllib/Logic and Bit Operations/Bit Shift  mode=Shift Right Arithmetic  N=4
  Bit Shift3 : hdlsllib/Logic and Bit Operations/Bit Shift  mode=Shift Right Arithmetic  N=8
  Bit Shift4 : hdlsllib/Logic and Bit Operations/Bit Shift  mode=Shift Right Arithmetic  N=16
  Bit Shift5 : hdlsllib/Logic and Bit Operations/Bit Shift  mode=Shift Right Arithmetic  N=32
  Bit Shift6 : hdlsllib/Logic and Bit Operations/Bit Shift  mode=Shift Right Arithmetic  N=64
  Bit Shift7 : hdlsllib/Logic and Bit Operations/Bit Shift  mode=Shift Right Arithmetic  N=128
  Bit Slice1 : hdlsllib/Logic and Bit Operations/Bit Slice  lidx=0  ridx=0
      settings: LibrarySourceBlock=embreciprocals/Real Divide HDL Optimized/ForEach - Real Divide/Shift and cast to output type/Variable Right Shift/Bit Slice1
  Bit Slice2 : hdlsllib/Logic and Bit Operations/Bit Slice  lidx=1  ridx=1
      settings: LibrarySourceBlock=embreciprocals/Real Divide HDL Optimized/ForEach - Real Divide/Shift and cast to output type/Variable Right Shift/Bit Slice2
  Bit Slice3 : hdlsllib/Logic and Bit Operations/Bit Slice  lidx=2  ridx=2
      settings: LibrarySourceBlock=embreciprocals/Real Divide HDL Optimized/ForEach - Real Divide/Shift and cast to output type/Variable Right Shift/Bit Slice3
  Bit Slice4 : hdlsllib/Logic and Bit Operations/Bit Slice  lidx=3  ridx=3
      settings: LibrarySourceBlock=embreciprocals/Real Divide HDL Optimized/ForEach - Real Divide/Shift and cast to output type/Variable Right Shift/Bit Slice4
  Bit Slice5 : hdlsllib/Logic and Bit Operations/Bit Slice  lidx=4  ridx=4
      settings: LibrarySourceBlock=embreciprocals/Real Divide HDL Optimized/ForEach - Real Divide/Shift and cast to output type/Variable Right Shift/Bit Slice5
  Bit Slice6 : hdlsllib/Logic and Bit Operations/Bit Slice  lidx=5  ridx=5
      settings: LibrarySourceBlock=embreciprocals/Real Divide HDL Optimized/ForEach - Real Divide/Shift and cast to output type/Variable Right Shift/Bit Slice6
  Bit Slice7 : hdlsllib/Logic and Bit Operations/Bit Slice  lidx=6  ridx=6
      settings: LibrarySourceBlock=embreciprocals/Real Divide HDL Optimized/ForEach - Real Divide/Shift and cast to output type/Variable Right Shift/Bit Slice7
  Bit Slice8 : hdlsllib/Logic and Bit Operations/Bit Slice  lidx=7  ridx=7
      settings: LibrarySourceBlock=embreciprocals/Real Divide HDL Optimized/ForEach - Real Divide/Shift and cast to output type/Variable Right Shift/Bit Slice8
  Delay{,1..4} (5 alike) : Delay  DelayLength=1
  Switch{1..8} (8 alike) : Switch  Criteria=u2 ~= 0  OutDataTypeStr=fixdt(1, 39, 23)  SaturateOnIntegerOverflow=off  InputSameDT=off
  y : Outport  SampleTime=2e-08
  wires:
  rightShift/1 -> Bit Slice8/1, Bit Slice7/1, Bit Slice6/1, Bit Slice5/1, Bit Slice4/1, Bit Slice3/1, Bit Slice2/1, Bit Slice1/1
  x/1 -> Switch1/3, Bit Shift/1
  Bit Shift/1 -> Switch1/1
  Bit Shift1/1 -> Switch2/1
  Bit Shift2/1 -> Switch3/1
  Bit Shift3/1 -> Switch4/1
  Bit Shift4/1 -> Switch5/1
  Bit Shift5/1 -> Switch6/1
  Bit Shift6/1 -> Switch7/1
  Bit Shift7/1 -> Switch8/1
  Bit Slice1/1 -> Switch1/2
  Bit Slice2/1 -> Switch2/2
  Bit Slice3/1 -> Switch3/2
  Bit Slice4/1 -> Switch4/2
  Bit Slice5/1 -> Delay1/1
  Bit Slice6/1 -> Delay2/1
  Bit Slice7/1 -> Delay3/1
  Bit Slice8/1 -> Delay4/1
  Delay/1 -> Switch5/3, Bit Shift4/1
  Delay1/1 -> Switch5/2
  Delay2/1 -> Switch6/2
  Delay3/1 -> Switch7/2
  Delay4/1 -> Switch8/2
  Switch1/1 -> Switch2/3, Bit Shift1/1
  Switch2/1 -> Switch3/3, Bit Shift2/1
  Switch3/1 -> Switch4/3, Bit Shift3/1
  Switch4/1 -> Delay/1
  Switch5/1 -> Switch6/3, Bit Shift5/1
  Switch6/1 -> Switch7/3, Bit Shift6/1
  Switch7/1 -> Switch8/3, Bit Shift7/1
  Switch8/1 -> y/1

== matlab function gm_HDLRx_vs/full_rx/rx_demodulator_full/ofdm_separator/Real Divide HDL Optimized/ForEach - Real Divide_instance1/Shift and cast to output type/Cast to Union of Types/slutils_c1_Cast_to_Union_of_Types ==
  settings: fimath=hdlfimath
  data: Xref input; Cout output; Cin input
function Cout = castToUnionType(Xref,Cin)
    %castToUnionType Cast second input to union of the two types
    if (isfloat(Xref) && isfloat(Cin)) || (isFixed(Xref) && isFixed(Cin))
        T = fixed.internal.type.unionPrototype(Cin,Xref,...
        'RoundingMethod','Floor',...
        'OverflowAction','Wrap');
        Cout = cast(Cin,'like',T);
    else
        coder.internal.assert(false,'fixed:emblib:InputOutputMustBeAllFixedOrFloat');
    end
end

function t = isFixed(x)
    t = (isfi(x) || isa(x,'embedded.numerictype')) && isscalingbinarypoint(x) ...
        || isinteger(x);
end
